simulink model "reconfig_dev_2021a_analytique"  (R2021a)
settings: Solver=VariableStepAuto  StartTime=0.0  StopTime=tsim  RelTol=1e-3
InitFcn:
  | main
values from neighbouring files (symbols this model uses):
  drone_params = get_parameters(3)    [main.m]
  dt = 0.005    [main.m]
  g = 9.81    [main.m]
  gust_duration = 5    [main.m]
  gust_force = [0;0;0]    [main.m]
  gust_start = 8    [main.m]
  omega0 = [[0,0,0]',[0,0,0]',[0,0,0]']    [main.m]
  p0 = [[0,0,2]',[0,0,2]',[0,0,2]']    [main.m]
  q0 = [[1,0,0,0]',[1,0,0,0]',[1,0,0,0]']    [main.m]
  tsim = 20    [main.m]
  v0 = [[0,0,0]',[0,0,0]',[0,0,0]']    [main.m]
undefined symbols (not defined in the file or in its folder): SMC_attitude_control, SMC_position_control, SMC_sliding_var, Twisting_attitude_control, Twisting_position_control, Twisting_sliding_var
libraries: vrlib x1
settings Model: Creator=gbattaglia2021  LastModifiedBy=jcolombini2021

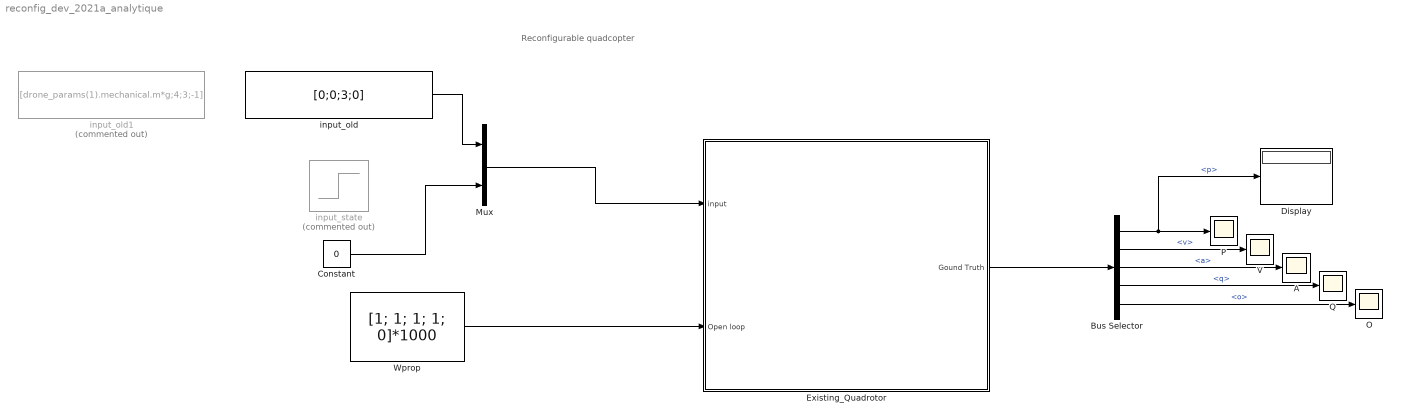
== system reconfig_dev_2021a_analytique ==
  note: Reconfigurable quadcopter
  "  Existing_Quadrotor" : Subsystem  mask{control_type_param=1: Position + Yaw, DroneID=1, DroneName=Drone1, idx_offset=0}
      mask prompts: control_type_param "Controller type"; DroneName "Drone Name"; idx_offset "Index Offset"
      mask TypeOptions control_type_param: 1: Position + Yaw | 2: Body Velocity + Yawrate | 3: Body Acceleration + Yawrate | 4: Thrust + Attitude | 5: Thrust + Body Rate | 6: Body Wrench
      mask TypeOptions DroneID: 1 | 2 | 3 | 4 | 5 | 6 | 7 | 8 | 9
      mask Callback DroneID:
      | ID = get_param(gcb,'DroneID');
      | offset = get_param(gcb,'idx_offset');
      | if ischar(ID)
      |   ID = str2num(ID);
      | end
      | if ischar(offset)
      |   offset = str2num(offset);
      | end
      | nameID = ID + offset;
      | set_param(gcb,'DroneName',["Drone"+num2str(nameID)]);
      mask Callback DroneName: set_param([gcb,'/To Workspace'],'VariableName',[get_param(gcb,'DroneName')]);
      mask Callback idx_offset:
      | ID = get_param(gcb,'DroneID');
      | offset = get_param(gcb,'idx_offset');
      | if ischar(ID)
      |   ID = str2num(ID);
      | end
      | if ischar(offset)
      |   offset = str2num(offset);
      | end
      | nameID = ID + offset;
      | set_param(gcb,'DroneName',["Drone"+num2str(nameID)]);
      mask DialogControl Control4 Prompt: click to choose controller
      mask Display:
      | image('format/drone_image.png'); % Use "Edit Image" on toolstrip to change.
      | Name = get_param(gcb,'DroneName');
      | ID = get_param(gcb,'DroneID');
      | C_mode = get_param(gcb,'control_type_param');
      | C_mode(1:2) = [];
      | color('red')
      | ID = "ID = "+ID;
      | color('red')
      | text(0.5, 0.25, Name, 'horizontalAlignment', 'center')
      | color('red')
      | text(0.5, 0.15, ID, 'horizontalAlignment', 'center')
      | color('blue');
      | text(0.5, 0.05, C_mode, 'horizontalAlignment', 'center')
  A : Scope
  Bus Selector : BusSelector  OutputSignals=p,v,a,q,o
  Constant : Constant  Value=0
  Display : Display
  Mux : Mux  Inputs=2
  O : Scope
  P : Scope
  Q : Scope
  V : Scope
  Wprop : Constant  Value=[1; 1; 1; 1; 0]*1000
  input_old : Constant  Value=[0;0;3;0]
  input_old1 : Constant  Commented=on  Value=[drone_params(1).mechanical.m*g;4;3;-1]
  input_state : Step  Commented=on  Time=tsim/2  Before=drone_params(1).control.state  After=drone_params(1).control.state_enum.folded2  SampleTime=0
  wires:
  Bus Selector/1 -> Display/1, P/1  "<p>"
  Bus Selector/4 -> Q/1  "<q>"
  Bus Selector/5 -> O/1  "<o>"
  Bus Selector/2 -> V/1  "<v>"
  "  Existing_Quadrotor"/1(Gound Truth) -> Bus Selector/1
  Bus Selector/3 -> A/1  "<a>"
  Wprop/1 -> "  Existing_Quadrotor"/2(Open loop)
  input_old/1 -> Mux/1
  Mux/1 -> "  Existing_Quadrotor"/1(input)
  Constant/1 -> Mux/2

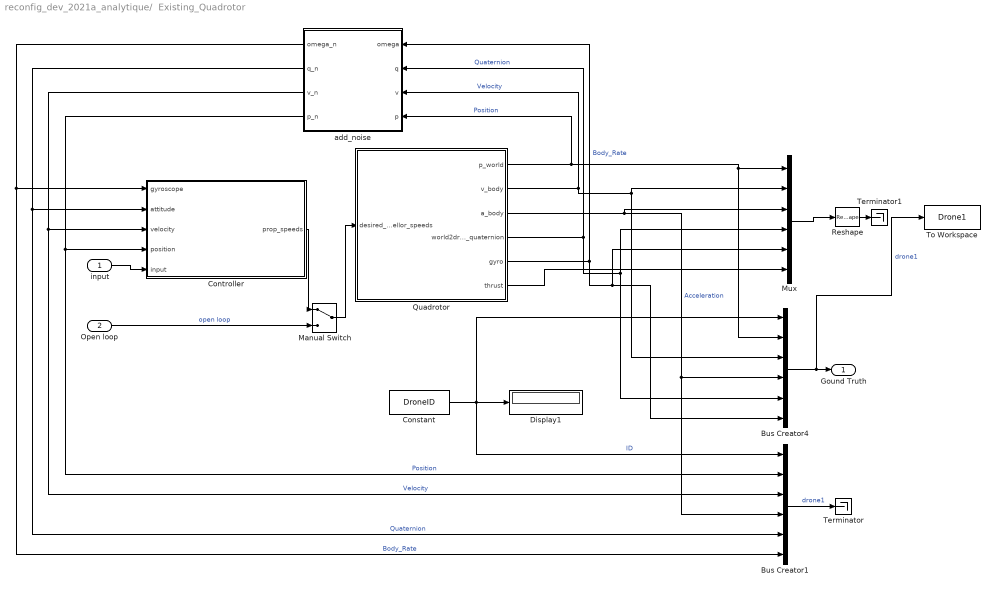
== system reconfig_dev_2021a_analytique/  Existing_Quadrotor ==
  input : Inport
  Open loop : Inport  Port=2
  Bus Creator1 : BusCreator  Inputs=6  OutDataTypeStr=Bus: DroneStateBus
      settings: InheritFromInputs=off
  Bus Creator4 : BusCreator  Inputs=6  OutDataTypeStr=Bus: DroneStateBus
      settings: InheritFromInputs=off
  Constant : Constant  Value=DroneID
  Controller : Subsystem
  Display1 : Display
  Manual Switch : ManualSwitch
  Mux : Mux  Inputs=6
  Quadrotor : Subsystem
      mask Display: image('droneHardware.jpeg'); % Use "Edit Image" on toolstrip to change.
  Reshape : Reshape
  Terminator : Terminator
  Terminator1 : Terminator
  To Workspace : ToWorkspace  VariableName=Drone1  SaveFormat=Timeseries  SampleTime=-1
  add_noise : MATLAB Function  TreatAsAtomicUnit=on
  Gound Truth : Outport
  wires:
  Quadrotor/5(gyro) -> add_noise/1(omega), Bus Creator4/6, Mux/5  "Body_Rate"
  Quadrotor/1(p_world) -> add_noise/4(p), Bus Creator4/2, Mux/1  "Position"
  Quadrotor/4(world2drone_quaternion) -> add_noise/2(q), Bus Creator4/5, Mux/4  "Quaternion"
  Mux/1 -> Reshape/1
  Quadrotor/2(v_body) -> add_noise/3(v), Bus Creator4/3, Mux/2  "Velocity"
  Quadrotor/6(thrust) -> Mux/6
  input/1 -> Controller/5(input)
  Bus Creator4/1 -> To Workspace/1, Gound Truth/1  "drone1"
  add_noise/2(q_n) -> Bus Creator1/5, Controller/2(attitude)  "Quaternion"
  Quadrotor/3(a_body) -> Mux/3, Bus Creator4/4, Bus Creator1/4  "Acceleration"
  Bus Creator1/1 -> Terminator/1  "drone1"
  add_noise/4(p_n) -> Bus Creator1/2, Controller/4(position)  "Position"
  add_noise/3(v_n) -> Bus Creator1/3, Controller/3(velocity)  "Velocity"
  Constant/1 -> Bus Creator4/1, Display1/1, Bus Creator1/1  "ID"
  add_noise/1(omega_n) -> Bus Creator1/6, Controller/1(gyroscope)  "Body_Rate"
  Reshape/1 -> Terminator1/1
  Manual Switch/1 -> Quadrotor/1(desired_propellor_speeds)
  Controller/1(prop_speeds) -> Manual Switch/1
  Open loop/1 -> Manual Switch/2  "open loop"

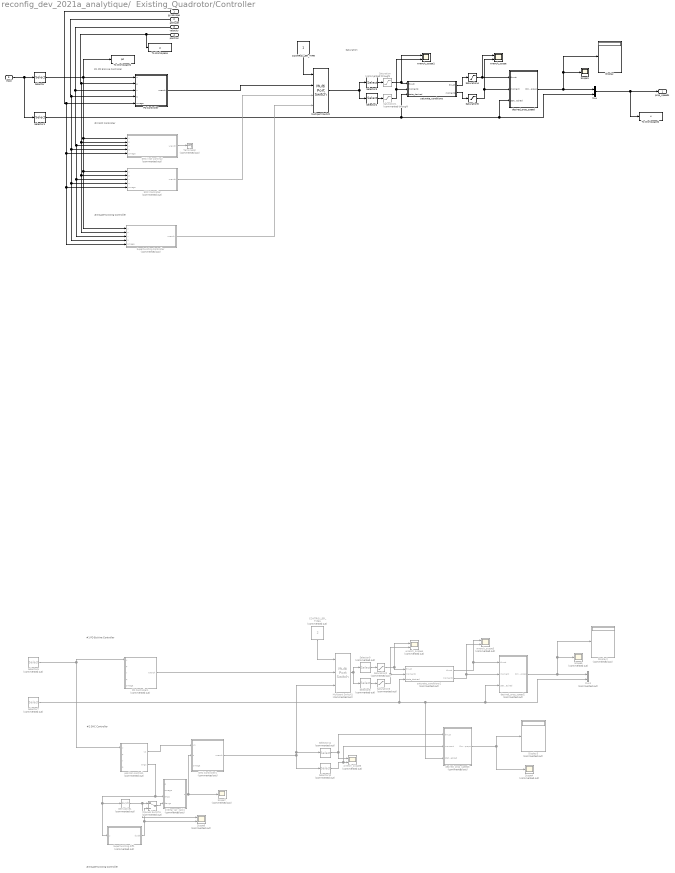
== system reconfig_dev_2021a_analytique/  Existing_Quadrotor/Controller ==
  note: Saturation
  note: #3 Supertwisting Controller
  note: #2 SMC Controller
  note: #1 PD Erskine Controller
  note: #3 Supertwisting Controller
  note: #1 PD Erskine Controller
  note: #2 SMC Controller
  gyroscope : Inport
  attitude : Inport  Port=2
  velocity : Inport  Port=3
  position : Inport  Port=4
  input : Inport  Port=5
  CONTROLLER_TYPE : Constant
  CONTROLLER_TYPE1 : Constant  Commented=on  Value=2
  Derivative1 : Derivative  Commented=on  CoefficientInTFapproximation=1000
  Display : Display
  Display2 : Display  Commented=on
  Display3 : Display  Commented=on
  Manual Switch1 : ManualSwitch  Commented=on
  Multiport Switch : MultiPortSwitch
  Multiport Switch1 : MultiPortSwitch  Commented=on  Inputs=2
  Mux : Mux  Inputs=2
  Mux1 : Mux  Commented=on  Inputs=2
  PD Controller : MATLAB Function  TreatAsAtomicUnit=on
  PD Controller1 : MATLAB Function  Commented=on  TreatAsAtomicUnit=on
  SMC (not working) : Subsystem  Commented=on
  SMC Controller : Subsystem  Commented=on
  SMC Controller1 : MATLAB Function  Commented=on  TreatAsAtomicUnit=on
  Saturation : Saturate  Commented=through  UpperLimit=16  LowerLimit=3
  Saturation1 : Saturate  Commented=through  UpperLimit=0.1  LowerLimit=-0.1
  Saturation2 : Saturate  Commented=on  UpperLimit=16  LowerLimit=3
  Saturation3 : Saturate  Commented=on  UpperLimit=0.1  LowerLimit=-0.1
  Saturation4 : Saturate  UpperLimit=16  LowerLimit=3
  Saturation5 : Saturate  UpperLimit=0.1  LowerLimit=-0.1
  Scope1 : Scope
  Scope4 : Scope  Commented=on
  Scope5 : Scope  Commented=on
  Scope6 : Scope  Commented=on  NumInputPorts=2
  Scope7 : Scope  Commented=on
  Selector : Selector  InputPortWidth=5  IndexOptions=Index vector (dialog)  Indices=[1 2 3 4]  OutputSizes=1
  Selector1 : Selector  InputPortWidth=5  IndexOptions=Index vector (dialog)  Indices=[5]  OutputSizes=1
  Selector10 : Selector  Commented=on  InputPortWidth=4  IndexOptions=Index vector (dialog)  Indices=[2 3 4]  OutputSizes=1
  Selector11 : Selector  Commented=on  InputPortWidth=4  IndexOptions=Index vector (dialog)  Indices=[1]  OutputSizes=1
  Selector2 : Selector  InputPortWidth=4  IndexOptions=Index vector (dialog)  Indices=[2 3 4]  OutputSizes=1
  Selector3 : Selector  InputPortWidth=4  IndexOptions=Index vector (dialog)  Indices=[1]  OutputSizes=1
  Selector6 : Selector  Commented=on  InputPortWidth=5  IndexOptions=Index vector (dialog)  Indices=[1 2 3 4]  OutputSizes=1
  Selector7 : Selector  Commented=on  InputPortWidth=5  IndexOptions=Index vector (dialog)  Indices=[5]  OutputSizes=1
  Selector8 : Selector  Commented=on  InputPortWidth=4  IndexOptions=Index vector (dialog)  Indices=[2 3 4]  OutputSizes=1
  Selector9 : Selector  Commented=on  InputPortWidth=4  IndexOptions=Index vector (dialog)  Indices=[1]  OutputSizes=1
  Supertwisting Controller : Subsystem  Commented=on
  Supertwisting diff1 : Subsystem  Commented=on
  Terminator : Terminator  Commented=on
  To Workspace : ToWorkspace  VariableName=p  SaveFormat=Timeseries  SampleTime=-1
  To Workspace1 : ToWorkspace  VariableName=pd  SaveFormat=Timeseries  SampleTime=-1
  To Workspace2 : ToWorkspace  VariableName=u  SaveFormat=Timeseries  SampleTime=-1
  desired_prop_speed : MATLAB Function  TreatAsAtomicUnit=on
  desired_prop_speed2 : MATLAB Function  Commented=on  TreatAsAtomicUnit=on
  desired_prop_speed3 : MATLAB Function  Commented=on  TreatAsAtomicUnit=on
  posiiton control1 : MATLAB Function  Commented=on  TreatAsAtomicUnit=on
  saturate_conditions : MATLAB Function  TreatAsAtomicUnit=on
  saturate_conditions1 : MATLAB Function  Commented=on  TreatAsAtomicUnit=on
  sliding_var_calc1 : MATLAB Function  Commented=on  TreatAsAtomicUnit=on
  wrench_scope : Scope  NumInputPorts=2
  wrench_scope1 : Scope  NumInputPorts=2
  wrench_scope3 : Scope  Commented=on  NumInputPorts=2
  wrench_scope4 : Scope  Commented=on  NumInputPorts=2
  wrench_scope5 : Scope  Commented=on  NumInputPorts=2
  prop_speeds : Outport
  wires:
  Saturation/1 -> wrench_scope1/1, saturate_conditions/1("thrust ")
  Saturation1/1 -> saturate_conditions/2("moments "), wrench_scope1/2
  Selector1/1 -> desired_prop_speed/3(state_desired), Mux/2, saturate_conditions/3(state_desired)
  input/1 -> Selector1/1, Selector/1
  Mux/1 -> To Workspace2/1, prop_speeds/1
  Selector2/1 -> Saturation1/1
  CONTROLLER_TYPE/1 -> Multiport Switch/1
  PD Controller/1(wrench) -> Multiport Switch/2
  Multiport Switch/1 -> Selector3/1, Selector2/1
  Selector3/1 -> Saturation/1
  desired_prop_speed/1(Omega_props) -> Mux/1, Scope1/1, Display/1
  Selector7/1 -> saturate_conditions1/3(state_desired), desired_prop_speed3/3(state_desired), desired_prop_speed2/3(state_desired), Mux1/2
  desired_prop_speed2/1(Omega_props) -> Mux1/1, Scope5/1, Display2/1
  Selector10/1 -> desired_prop_speed3/2(moment), wrench_scope5/2
  Manual Switch1/1 -> sliding_var_calc1/4(dangc)
  Selector11/1 -> wrench_scope5/1, desired_prop_speed3/1(thrust)
  CONTROLLER_TYPE1/1 -> Multiport Switch1/1
  Selector6/1 -> posiiton control1/1(u), PD Controller1/1(u)
  SMC Controller1/1(wrench) -> Selector10/1, Selector11/1, Multiport Switch1/3
  posiiton control1/2(angc) -> sliding_var_calc1/3(angc), Derivative1/1, Supertwisting diff1/1(u)
  Derivative1/1 -> Scope6/1, Manual Switch1/1
  PD Controller1/1(wrench) -> Multiport Switch1/2
  Multiport Switch1/1 -> Selector9/1, Selector8/1
  Selector8/1 -> Saturation3/1
  sliding_var_calc1/1(s) -> Scope7/1, SMC Controller1/2(s)
  Supertwisting diff1/1(du/dt) -> Manual Switch1/2, Scope6/2
  Saturation3/1 -> saturate_conditions1/2("moments "), wrench_scope4/2
  posiiton control1/1(u1) -> SMC Controller1/1(u1)
  Selector9/1 -> Saturation2/1
  desired_prop_speed3/1(Omega_props) -> Scope4/1, Display3/1
  Saturation2/1 -> wrench_scope4/1, saturate_conditions1/1("thrust ")
  saturate_conditions1/1(thrust) -> desired_prop_speed2/1(thrust), wrench_scope3/1
  saturate_conditions1/2(moments) -> desired_prop_speed2/2(moment), wrench_scope3/2
  saturate_conditions/2(moments) -> Saturation5/1
  Saturation4/1 -> wrench_scope/1, desired_prop_speed/1(thrust)
  Saturation5/1 -> wrench_scope/2, desired_prop_speed/2(moment)
  saturate_conditions/1(thrust) -> Saturation4/1
  Selector/1 -> To Workspace1/1, Supertwisting Controller/1(u), SMC Controller/1(u), SMC (not working)/1(u), PD Controller/1(u)
  gyroscope/1 -> PD Controller/5(omega), Supertwisting Controller/5(omega), SMC Controller/5(omega), SMC (not working)/5(omega)
  position/1 -> To Workspace/1, PD Controller/2(p), SMC (not working)/2(p), Supertwisting Controller/2(p), SMC Controller/2(p)
  velocity/1 -> PD Controller/3(v), Supertwisting Controller/3("v "), SMC Controller/3("v "), SMC (not working)/3(v)
  attitude/1 -> Supertwisting Controller/4(q), SMC Controller/4(q), SMC (not working)/4(q), PD Controller/4(q)
  SMC Controller/1(wrench) -> Multiport Switch/3
  Supertwisting Controller/1(wrench) -> Multiport Switch/4
  SMC (not working)/1(wrench) -> Terminator/1

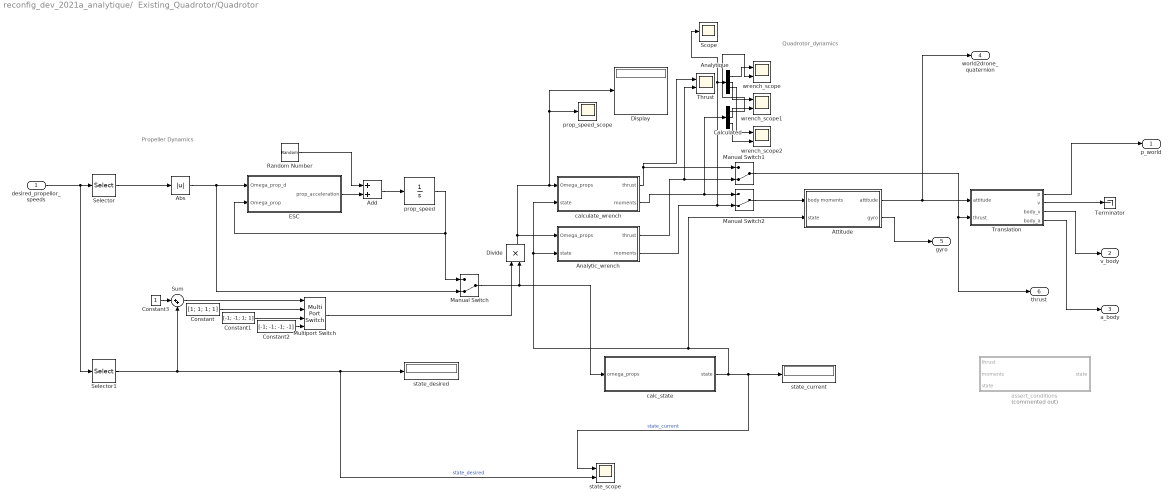
== system reconfig_dev_2021a_analytique/  Existing_Quadrotor/Quadrotor ==
  note: Quadrotor_dynamics
  note: Propeller Dynamics
  desired_propellor_speeds : Inport
  Abs : Abs
  Add : Sum
  Analytic_wrench : MATLAB Function  TreatAsAtomicUnit=on
  Analytique : Demux  Outputs=3
  Attitude : Subsystem
  Calculated : Demux  Outputs=3
  Constant : Constant  Value=[1; 1; 1; 1]
  Constant1 : Constant  Value=[-1; -1; 1; 1]
  Constant2 : Constant  Value=[-1; -1; -1; -1]
  Constant3 : Constant
  Display : Display
  Divide : Product
  ESC : MATLAB Function  TreatAsAtomicUnit=on
  Manual Switch : ManualSwitch  CurrentSetting=0
  Manual Switch1 : ManualSwitch  CurrentSetting=0
  Manual Switch2 : ManualSwitch  CurrentSetting=0
  Multiport Switch : MultiPortSwitch
  Random Number : RandomNumber  Mean=[0;0;0;0]  Variance=[5000;5000;5000;5000]  Seed=[1;2;3;4]  SampleTime=dt
  Scope : Scope
  Selector : Selector  InputPortWidth=5  IndexOptions=Index vector (dialog)  Indices=[1 2 3 4]  OutputSizes=1
  Selector1 : Selector  InputPortWidth=5  IndexOptions=Index vector (dialog)  Indices=[5]  OutputSizes=1
  Sum : Sum  Inputs=|++
  Terminator : Terminator
  Thrust : Scope  NumInputPorts=2
  Translation : Subsystem
  assert_conditions : MATLAB Function  Commented=on  TreatAsAtomicUnit=on
  calc_state : MATLAB Function  TreatAsAtomicUnit=on
  calculate_wrench : MATLAB Function  TreatAsAtomicUnit=on
  prop_speed : Integrator  InitialCondition=drone_params(DroneID).motors.omega0  LimitOutput=on  UpperSaturationLimit=drone_params(DroneID).motors.omega_max  LowerSaturationLimit=drone_params(DroneID).motors.omega_min
  prop_speed_scope : Scope
  state_current : Display
  state_desired : Display
  state_scope : Scope  NumInputPorts=2
  wrench_scope : Scope  NumInputPorts=2
  wrench_scope1 : Scope  NumInputPorts=2
  wrench_scope2 : Scope  NumInputPorts=2
  p_world : Outport
  v_body : Outport  Port=2
  a_body : Outport  Port=3
  world2drone_quaternion : Outport  Port=4
  gyro : Outport  Port=5
  thrust : Outport  Port=6
  wires:
  calculate_wrench/1(thrust) -> Thrust/1, Manual Switch1/1
  Add/1 -> prop_speed/1
  desired_propellor_speeds/1 -> Selector1/1, Selector/1
  prop_speed/1 -> Manual Switch/1, ESC/2(Omega_prop)
  calculate_wrench/2(moments) -> Manual Switch2/1, Calculated/1
  Attitude/1(attitude) -> world2drone_quaternion/1, Translation/1(attitude)
  Attitude/2(gyro) -> gyro/1
  Translation/3(body_v) -> v_body/1
  Translation/4(body_a) -> a_body/1
  Translation/1(p) -> p_world/1
  Random Number/1 -> Add/1
  ESC/1(prop_acceleration) -> Add/2
  Manual Switch/1 -> calc_state/1(omega_props), Divide/2
  Translation/2(v) -> Terminator/1
  Abs/1 -> Manual Switch/2, ESC/1(Omega_prop_d)
  Selector1/1 -> state_scope/2, state_desired/1, Sum/2  "state_desired"
  calc_state/1(state) -> state_scope/1, state_current/1, Analytic_wrench/2(state), calculate_wrench/2(state), Attitude/2(state)  "state_current"
  Selector/1 -> Abs/1
  Multiport Switch/1 -> Divide/1
  Divide/1 -> Analytic_wrench/1(Omega_props), Display/1, prop_speed_scope/1, calculate_wrench/1(Omega_props)
  Constant3/1 -> Sum/1
  Sum/1 -> Multiport Switch/1
  Constant/1 -> Multiport Switch/2
  Constant1/1 -> Multiport Switch/3
  Constant2/1 -> Multiport Switch/4
  Analytic_wrench/1(thrust) -> Manual Switch1/2, Thrust/2
  Analytic_wrench/2(moments) -> Manual Switch2/2, Scope/1, Analytique/1
  Manual Switch1/1 -> thrust/1, Translation/2(thrust)
  Manual Switch2/1 -> Attitude/1(body moments)
  Analytique/1 -> wrench_scope/1
  Analytique/3 -> wrench_scope2/1
  Analytique/2 -> wrench_scope1/1
  Calculated/1 -> wrench_scope/2
  Calculated/2 -> wrench_scope1/2
  Calculated/3 -> wrench_scope2/2

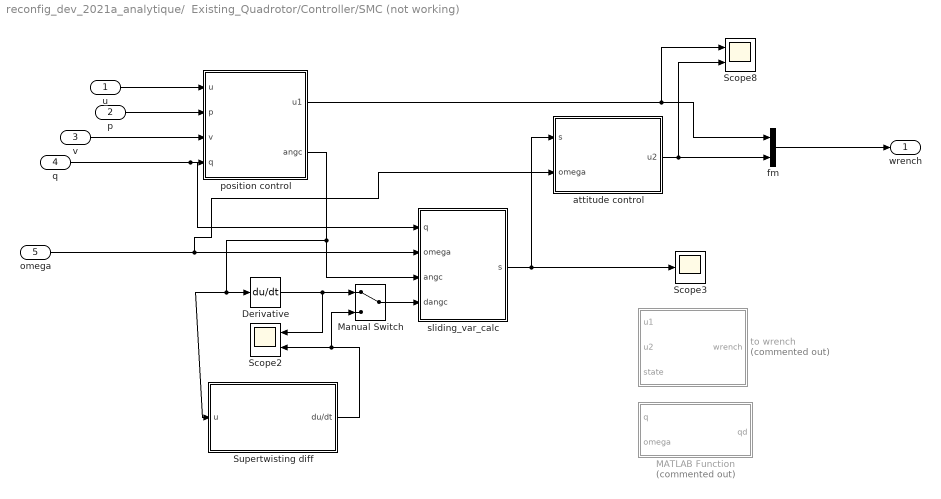
== system reconfig_dev_2021a_analytique/  Existing_Quadrotor/Controller/SMC (not working) ==
  u : Inport
  p : Inport  Port=2
  v : Inport  Port=3
  q : Inport  Port=4
  omega : Inport  Port=5
  Derivative : Derivative  CoefficientInTFapproximation=1000
  MATLAB Function : MATLAB Function  Commented=on  TreatAsAtomicUnit=on
  Manual Switch : ManualSwitch
  Scope2 : Scope  NumInputPorts=2
  Scope3 : Scope
  Scope8 : Scope  NumInputPorts=2
  Supertwisting diff : Subsystem
  attitude control : MATLAB Function  TreatAsAtomicUnit=on
  fm : Mux  Inputs=2
  position control : MATLAB Function  TreatAsAtomicUnit=on
  sliding_var_calc : MATLAB Function  TreatAsAtomicUnit=on
  to wrench : MATLAB Function  Commented=on  TreatAsAtomicUnit=on
  wrench : Outport
  wires:
  position control/2(angc) -> sliding_var_calc/3(angc), Supertwisting diff/1(u), Derivative/1
  position control/1(u1) -> fm/1, Scope8/1
  Supertwisting diff/1(du/dt) -> Manual Switch/2, Scope2/2
  Derivative/1 -> Manual Switch/1, Scope2/1
  q/1 -> position control/4(q), sliding_var_calc/1(q)
  attitude control/1(u2) -> fm/2, Scope8/2
  sliding_var_calc/1(s) -> Scope3/1, attitude control/1(s)
  v/1 -> position control/3(v)
  omega/1 -> attitude control/2(omega), sliding_var_calc/2(omega)
  Manual Switch/1 -> sliding_var_calc/4(dangc)
  fm/1 -> wrench/1
  p/1 -> position control/2(p)
  u/1 -> position control/1(u)

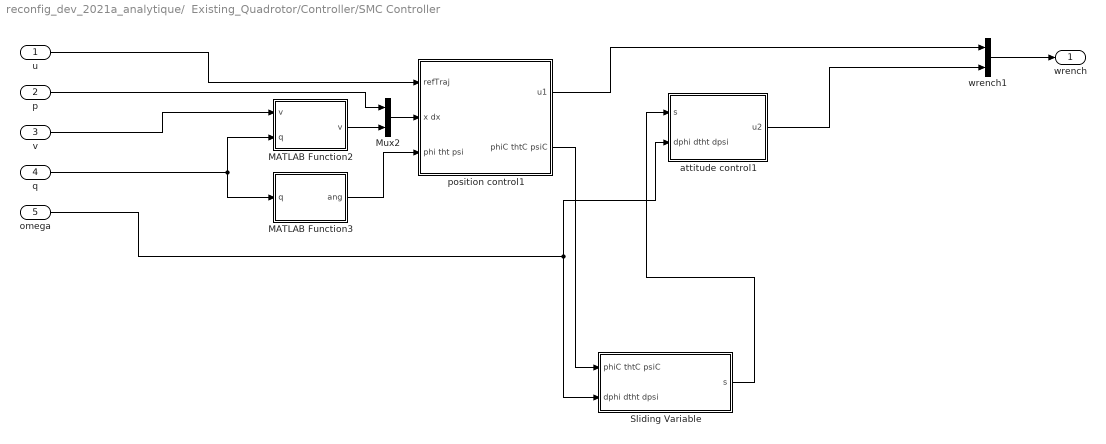
== system reconfig_dev_2021a_analytique/  Existing_Quadrotor/Controller/SMC Controller ==
  u : Inport
  p : Inport  Port=2
  "v " : Inport  Port=3
  q : Inport  Port=4
  omega : Inport  Port=5
  MATLAB Function2 : MATLAB Function  TreatAsAtomicUnit=on
  MATLAB Function3 : MATLAB Function  TreatAsAtomicUnit=on
  Mux2 : Mux  Inputs=2
  Sliding Variable : Subsystem
  attitude control1 : Subsystem
  position control1 : Subsystem
  wrench1 : Mux  Inputs=2
  wrench : Outport
  wires:
  position control1/2(phiC thtC psiC) -> Sliding Variable/1(phiC thtC psiC)
  q/1 -> MATLAB Function2/2(q), MATLAB Function3/1(q)
  p/1 -> Mux2/1
  attitude control1/1(u2) -> wrench1/2
  Sliding Variable/1(s) -> attitude control1/1(s)
  MATLAB Function2/1(v) -> Mux2/2
  Mux2/1 -> position control1/2(x dx)
  omega/1 -> attitude control1/2(dphi dtht dpsi), Sliding Variable/2(dphi dtht dpsi)
  position control1/1(u1) -> wrench1/1
  MATLAB Function3/1(ang) -> position control1/3(phi tht psi)
  wrench1/1 -> wrench/1
  u/1 -> position control1/1(refTraj)
  "v "/1 -> MATLAB Function2/1("v ")

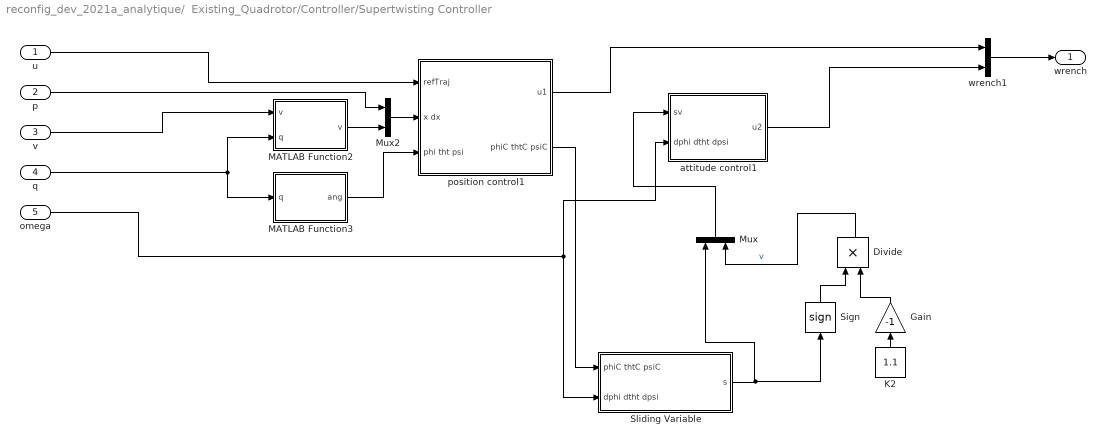
== system reconfig_dev_2021a_analytique/  Existing_Quadrotor/Controller/Supertwisting Controller ==
  u : Inport
  p : Inport  Port=2
  "v " : Inport  Port=3
  q : Inport  Port=4
  omega : Inport  Port=5
  Divide : Product
  Gain : Gain  Gain=-1
  K2 : Constant  Value=1.1
  MATLAB Function2 : MATLAB Function  TreatAsAtomicUnit=on
  MATLAB Function3 : MATLAB Function  TreatAsAtomicUnit=on
  Mux : Mux  Inputs=2
  Mux2 : Mux  Inputs=2
  Sign : Signum
  Sliding Variable : Subsystem
  attitude control1 : Subsystem
  position control1 : Subsystem
  wrench1 : Mux  Inputs=2
  wrench : Outport
  wires:
  position control1/2(phiC thtC psiC) -> Sliding Variable/1(phiC thtC psiC)
  q/1 -> MATLAB Function2/2(q), MATLAB Function3/1(q)
  p/1 -> Mux2/1
  attitude control1/1(u2) -> wrench1/2
  MATLAB Function2/1(v) -> Mux2/2
  Mux2/1 -> position control1/2(x dx)
  omega/1 -> attitude control1/2(dphi dtht dpsi), Sliding Variable/2(dphi dtht dpsi)
  position control1/1(u1) -> wrench1/1
  MATLAB Function3/1(ang) -> position control1/3(phi tht psi)
  wrench1/1 -> wrench/1
  u/1 -> position control1/1(refTraj)
  "v "/1 -> MATLAB Function2/1("v ")
  Sliding Variable/1(s) -> Sign/1, Mux/1
  Mux/1 -> attitude control1/1(sv)
  K2/1 -> Gain/1
  Sign/1 -> Divide/1
  Gain/1 -> Divide/2
  Divide/1 -> Mux/2  "v"

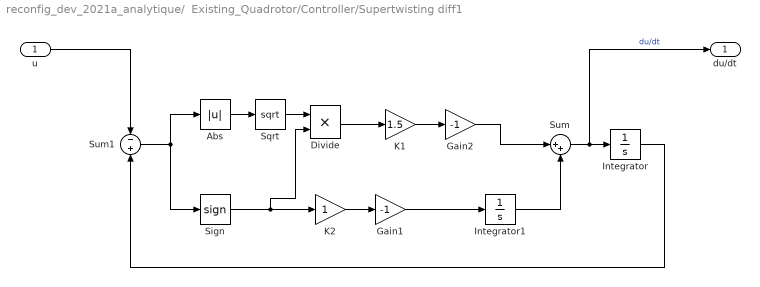
== system reconfig_dev_2021a_analytique/  Existing_Quadrotor/Controller/Supertwisting diff1 ==
  u : Inport
  Abs : Abs
  Divide : Product
  Gain1 : Gain  Gain=-1
  Gain2 : Gain  Gain=-1
  Integrator : Integrator  InitialCondition=[0;0;0]
  Integrator1 : Integrator  InitialCondition=[0;0;0]
  K1 : Gain  Gain=1.5
  K2 : Gain
  Sign : Signum
  Sqrt : Sqrt  SaturateOnIntegerOverflow=on
  Sum : Sum  Inputs=|++
  Sum1 : Sum  Inputs=-+
  du/dt : Outport
  wires:
  Integrator1/1 -> Sum/2
  Integrator/1 -> Sum1/2
  K1/1 -> Gain2/1
  Sum/1 -> du/dt/1, Integrator/1  "du/dt"
  Sum1/1 -> Sign/1, Abs/1
  Gain1/1 -> Integrator1/1
  K2/1 -> Gain1/1
  Abs/1 -> Sqrt/1
  Gain2/1 -> Sum/1
  Sign/1 -> Divide/2, K2/1
  Divide/1 -> K1/1
  Sqrt/1 -> Divide/1
  u/1 -> Sum1/1

== system reconfig_dev_2021a_analytique/  Existing_Quadrotor/Quadrotor/Attitude ==
  body moments : Inport
  state : Inport  Port=2
  Attitude : Integrator  InitialCondition=q0(:,DroneID)
  MATLAB Function : MATLAB Function  TreatAsAtomicUnit=on
  MATLAB Function1 : MATLAB Function  TreatAsAtomicUnit=on
  Normalize Vector : vrlib/Utilities/Normalize Vector  maxzero=0
  Sine Wave : Sin  Commented=on  Amplitude=[0.5;0.5;0.5]  Frequency=[1;0.3;0.6]  SampleTime=0
  angular velocity : Integrator  InitialCondition=omega0(:,DroneID)
  attitude : Outport
  gyro : Outport  Port=2
  wires:
  Attitude/1 -> Normalize Vector/1
  MATLAB Function/1(qd) -> Attitude/1  "quaternion derivative"
  body moments/1 -> MATLAB Function1/1(m)
  MATLAB Function1/1(a) -> angular velocity/1  "body angular acceleration"
  angular velocity/1 -> gyro/1, MATLAB Function/2(omega), MATLAB Function1/2(omega)  "gyroscope"
  Normalize Vector/1 -> MATLAB Function/1(q), attitude/1  "unit quaternion"
  state/1 -> MATLAB Function1/3(state)

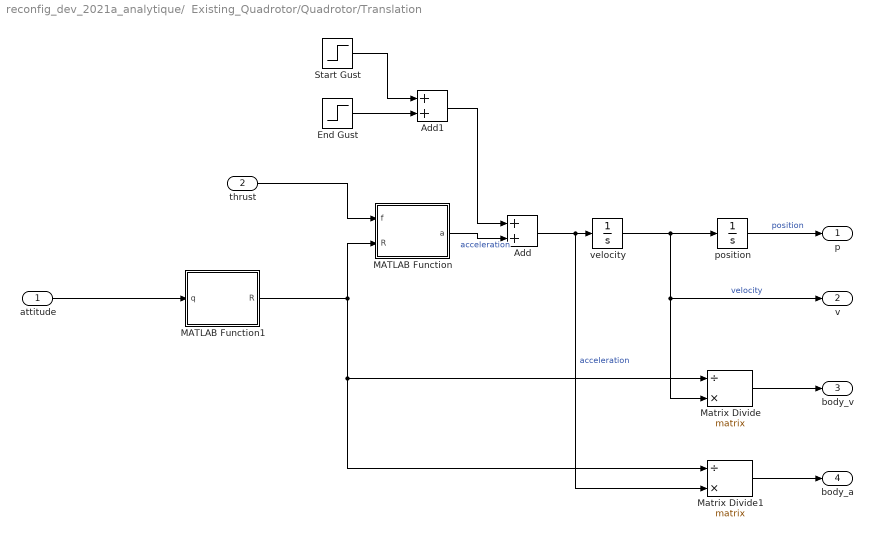
== system reconfig_dev_2021a_analytique/  Existing_Quadrotor/Quadrotor/Translation ==
  attitude : Inport
  thrust : Inport  Port=2
  Add : Sum
  Add1 : Sum
  End Gust : Step  Time=gust_start + gust_duration  Before=[0;0;0]  After=-1*gust_force/drone_params(DroneID).mechanical.m  SampleTime=0
  MATLAB Function : MATLAB Function  TreatAsAtomicUnit=on
  MATLAB Function1 : MATLAB Function  TreatAsAtomicUnit=on
  Matrix Divide : Product  Inputs=/*  Multiplication=Matrix(*)
  Matrix Divide1 : Product  Inputs=/*  Multiplication=Matrix(*)
  Start Gust : Step  Time=gust_start  Before=[0;0;0]  After=gust_force/drone_params(DroneID).mechanical.m  SampleTime=0
  position : Integrator  InitialCondition=p0(:,DroneID)
  velocity : Integrator  InitialCondition=v0(:,DroneID)
  p : Outport
  v : Outport  Port=2
  body_v : Outport  Port=3
  body_a : Outport  Port=4
  wires:
  velocity/1 -> Matrix Divide/2, v/1, position/1  "velocity"
  position/1 -> p/1  "position"
  Add/1 -> Matrix Divide1/2, velocity/1  "acceleration"
  attitude/1 -> MATLAB Function1/1(q)
  thrust/1 -> MATLAB Function/1(f)
  MATLAB Function1/1(R) -> Matrix Divide1/1, Matrix Divide/1, MATLAB Function/2(R)
  Matrix Divide/1 -> body_v/1
  Matrix Divide1/1 -> body_a/1
  MATLAB Function/1(a) -> Add/2  "acceleration"
  Add1/1 -> Add/1
  End Gust/1 -> Add1/2
  Start Gust/1 -> Add1/1

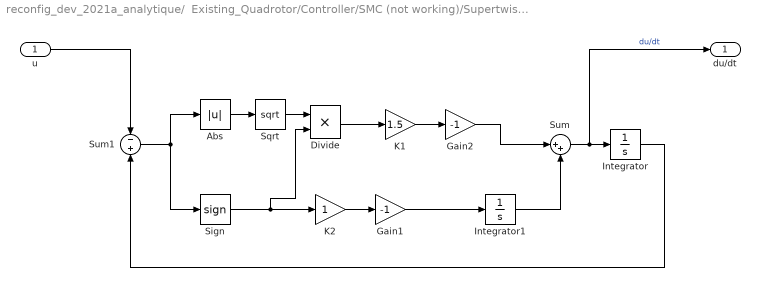
== system reconfig_dev_2021a_analytique/  Existing_Quadrotor/Controller/SMC (not working)/Supertwisting diff ==
  u : Inport
  Abs : Abs
  Divide : Product
  Gain1 : Gain  Gain=-1
  Gain2 : Gain  Gain=-1
  Integrator : Integrator  InitialCondition=[0;0;0]
  Integrator1 : Integrator  InitialCondition=[0;0;0]
  K1 : Gain  Gain=1.5
  K2 : Gain
  Sign : Signum
  Sqrt : Sqrt  SaturateOnIntegerOverflow=on
  Sum : Sum  Inputs=|++
  Sum1 : Sum  Inputs=-+
  du/dt : Outport
  wires:
  Integrator1/1 -> Sum/2
  Integrator/1 -> Sum1/2
  K1/1 -> Gain2/1
  Sum/1 -> du/dt/1, Integrator/1  "du/dt"
  Sum1/1 -> Sign/1, Abs/1
  Gain1/1 -> Integrator1/1
  K2/1 -> Gain1/1
  Abs/1 -> Sqrt/1
  Gain2/1 -> Sum/1
  Sign/1 -> Divide/2, K2/1
  Divide/1 -> K1/1
  Sqrt/1 -> Divide/1
  u/1 -> Sum1/1

== system reconfig_dev_2021a_analytique/  Existing_Quadrotor/Controller/SMC Controller/Sliding Variable ==
  phiC thtC psiC : Inport
  dphi dtht dpsi : Inport  Port=2
  Derivative : Derivative
  Integrator2 : Integrator
  Interpreted MATLAB Function : MATLABFcn  MATLABFcn=SMC_sliding_var(u)  OutputDimensions=3
  Mux2 : Mux
  s : Outport
  wires:
  Integrator2/1 -> Mux2/2
  Mux2/1 -> Interpreted MATLAB Function/1
  dphi dtht dpsi/1 -> Integrator2/1, Mux2/1
  Interpreted MATLAB Function/1 -> s/1
  phiC thtC psiC/1 -> Derivative/1, Mux2/3
  Derivative/1 -> Mux2/4

== system reconfig_dev_2021a_analytique/  Existing_Quadrotor/Controller/SMC Controller/attitude control1 ==
  s : Inport
  dphi dtht dpsi : Inport  Port=2
  Interpreted MATLAB Function : MATLABFcn  MATLABFcn=SMC_attitude_control(u)  OutputDimensions=3
  Mux : Mux  Inputs=2
  u2 : Outport
  wires:
  Mux/1 -> Interpreted MATLAB Function/1
  Interpreted MATLAB Function/1 -> u2/1
  dphi dtht dpsi/1 -> Mux/1
  s/1 -> Mux/2

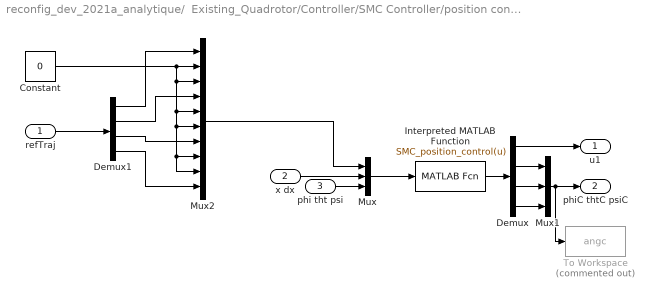
== system reconfig_dev_2021a_analytique/  Existing_Quadrotor/Controller/SMC Controller/position control1 ==
  refTraj : Inport
  x dx : Inport  Port=2
  phi tht psi : Inport  Port=3
  Constant : Constant  Value=0
  Demux : Demux
  Demux1 : Demux
  Interpreted MATLAB Function : MATLABFcn  MATLABFcn=SMC_position_control(u)  OutputDimensions=4
  Mux : Mux  Inputs=3
  Mux1 : Mux  Inputs=3
  Mux2 : Mux  Inputs=10
  To Workspace : ToWorkspace  Commented=on  VariableName=angc  SampleTime=-1
  u1 : Outport
  phiC thtC psiC : Outport  Port=2
  wires:
  Mux/1 -> Interpreted MATLAB Function/1
  x dx/1 -> Mux/2
  phi tht psi/1 -> Mux/3
  Interpreted MATLAB Function/1 -> Demux/1
  Demux/1 -> u1/1
  Demux/2 -> Mux1/1
  Demux/3 -> Mux1/2
  Demux/4 -> Mux1/3
  Mux1/1 -> To Workspace/1, phiC thtC psiC/1
  Mux2/1 -> Mux/1
  Constant/1 -> Mux2/9, Mux2/8, Mux2/6, Mux2/5, Mux2/3, Mux2/2
  refTraj/1 -> Demux1/1
  Demux1/1 -> Mux2/1
  Demux1/2 -> Mux2/4
  Demux1/3 -> Mux2/7
  Demux1/4 -> Mux2/10

== system reconfig_dev_2021a_analytique/  Existing_Quadrotor/Controller/Supertwisting Controller/Sliding Variable ==
  phiC thtC psiC : Inport
  dphi dtht dpsi : Inport  Port=2
  Derivative : Derivative
  Integrator2 : Integrator
  Interpreted MATLAB Function : MATLABFcn  MATLABFcn=Twisting_sliding_var(u)  OutputDimensions=3
  Mux2 : Mux
  s : Outport
  wires:
  Integrator2/1 -> Mux2/2
  Mux2/1 -> Interpreted MATLAB Function/1
  dphi dtht dpsi/1 -> Integrator2/1, Mux2/1
  Interpreted MATLAB Function/1 -> s/1
  phiC thtC psiC/1 -> Derivative/1, Mux2/3
  Derivative/1 -> Mux2/4

== system reconfig_dev_2021a_analytique/  Existing_Quadrotor/Controller/Supertwisting Controller/attitude control1 ==
  sv : Inport
  dphi dtht dpsi : Inport  Port=2
  Interpreted MATLAB Function : MATLABFcn  MATLABFcn=Twisting_attitude_control(u)  OutputDimensions=3
  Mux : Mux  Inputs=2
  u2 : Outport
  wires:
  Mux/1 -> Interpreted MATLAB Function/1
  Interpreted MATLAB Function/1 -> u2/1
  dphi dtht dpsi/1 -> Mux/1
  sv/1 -> Mux/2

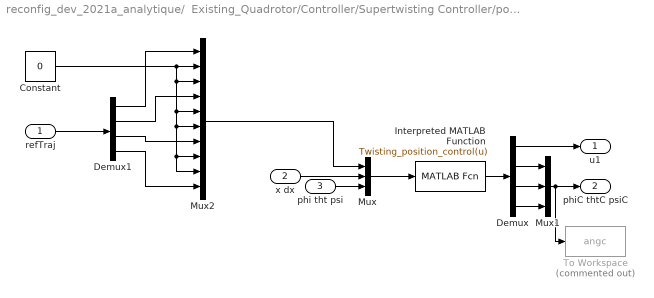
== system reconfig_dev_2021a_analytique/  Existing_Quadrotor/Controller/Supertwisting Controller/position control1 ==
  refTraj : Inport
  x dx : Inport  Port=2
  phi tht psi : Inport  Port=3
  Constant : Constant  Value=0
  Demux : Demux
  Demux1 : Demux
  Interpreted MATLAB Function : MATLABFcn  MATLABFcn=Twisting_position_control(u)  OutputDimensions=4
  Mux : Mux  Inputs=3
  Mux1 : Mux  Inputs=3
  Mux2 : Mux  Inputs=10
  To Workspace : ToWorkspace  Commented=on  VariableName=angc  SampleTime=-1
  u1 : Outport
  phiC thtC psiC : Outport  Port=2
  wires:
  Mux/1 -> Interpreted MATLAB Function/1
  x dx/1 -> Mux/2
  phi tht psi/1 -> Mux/3
  Interpreted MATLAB Function/1 -> Demux/1
  Demux/1 -> u1/1
  Demux/2 -> Mux1/1
  Demux/3 -> Mux1/2
  Demux/4 -> Mux1/3
  Mux1/1 -> To Workspace/1, phiC thtC psiC/1
  Mux2/1 -> Mux/1
  Constant/1 -> Mux2/9, Mux2/8, Mux2/6, Mux2/5, Mux2/3, Mux2/2
  refTraj/1 -> Demux1/1
  Demux1/1 -> Mux2/1
  Demux1/2 -> Mux2/4
  Demux1/3 -> Mux2/7
  Demux1/4 -> Mux2/10

== matlab function reconfig_dev_2021a_analytique/  Existing_Quadrotor/Controller/PD Controller1 ==
  data: u input; p input size=3; v input size=3; q input size=4; omega input size=3; wrench output size=4; control_type_param parameter; drone_params parameter; DroneID parameter; g parameter
function wrench = controller(u, p, v, q, omega, control_type_param, drone_params, DroneID, g)

    thrust = 1; % set output dim
    moments = [0;0;0]; % set output dim
    wrench = [0;0;0;0]; % set output dim

  coder.extrinsic('droneControl'); % link simulink to matlab function
  
  % do control
  [thrust, moments] = droneControl(u, p, v, q, omega, ...
    control_type_param, drone_params, DroneID, g);

  wrench = [thrust; moments];

end

== matlab function reconfig_dev_2021a_analytique/  Existing_Quadrotor/Controller/SMC Controller1 ==
  data: u1 input; s input size=3; omega input size=3; wrench output size=4; drone_params parameter; DroneID parameter
function wrench = controller(u1, s, omega, drone_params, DroneID)

%     thrust = 1; % set output dim
%     moments = [0;0;0]; % set output dim
    wrench = [0;0;0;0]; % set output dim

    coder.extrinsic('droneControlSMC'); % link simulink to matlab function
  
    % do control
    [thrust, moments] = droneControlSMC(u1, s, omega, ...
        drone_params, DroneID);

    wrench = [thrust; moments];

    
end

== matlab function reconfig_dev_2021a_analytique/  Existing_Quadrotor/Controller/desired_prop_speed2 ==
  data: thrust input; Omega_props output; moment input; state_desired input; drone_params parameter; DroneID parameter
function Omega_props  =  Allocation(thrust, moment, state_desired, drone_params, DroneID)

M = drone_params(DroneID).control.allocation_matrix;
if state_desired ~= drone_params(DroneID).control.state
switch state_desired
    case drone_params(DroneID).control.state_enum.unfolded
        M = drone_params(DroneID).control.allocation_matrix_u;
    case drone_params(DroneID).control.state_enum.folded2
        M = drone_params(DroneID).control.allocation_matrix_2f;
    case drone_params(DroneID).control.state_enum.folded4
        M = drone_params(DroneID).control.allocation_matrix_4f;
end
end

%  Omega_props = sqrt(inv(alloc_mat) * [thrust;moment]);
if state_desired ~= drone_params(DroneID).control.state_enum.folded4
    W2 = M \ [thrust;moment];
    Omega_props = real(sqrt(complex(W2)));
else
    W2 = pinv(M(2:4,:)) * moment;
    Omega_props = real(sqrt(complex(W2)));
end

if state_desired == drone_params(DroneID).control.state_enum.folded2
    Omega_props = Omega_props.*[-1; -1; 1; 1];
elseif state_desired == drone_params(DroneID).control.state_enum.folded4
    Omega_props = Omega_props.*[-1; -1; -1; -1];
end

== matlab function reconfig_dev_2021a_analytique/  Existing_Quadrotor/Controller/desired_prop_speed3 ==
  data: thrust input; Omega_props output; moment input; state_desired input; drone_params parameter; DroneID parameter
function Omega_props  =  Allocation(thrust, moment, state_desired, drone_params, DroneID)

M = drone_params(DroneID).control.allocation_matrix;
if state_desired ~= drone_params(DroneID).control.state
switch state_desired
    case drone_params(DroneID).control.state_enum.unfolded
        M = drone_params(DroneID).control.allocation_matrix_u;
    case drone_params(DroneID).control.state_enum.folded2
        M = drone_params(DroneID).control.allocation_matrix_2f;
    case drone_params(DroneID).control.state_enum.folded4
        M = drone_params(DroneID).control.allocation_matrix_4f;
end
end

%  Omega_props = sqrt(inv(alloc_mat) * [thrust;moment]);
if state_desired ~= drone_params(DroneID).control.state_enum.folded4
    W2 = M \ [thrust;moment];
    Omega_props = real(sqrt(complex(W2)));
else
    W2 = pinv(M(2:4,:)) * moment;
    Omega_props = real(sqrt(complex(W2)));
end

if state_desired == drone_params(DroneID).control.state_enum.folded2
    Omega_props = Omega_props.*[-1; -1; 1; 1];
elseif state_desired == drone_params(DroneID).control.state_enum.folded4
    Omega_props = Omega_props.*[-1; -1; -1; -1];
end

== matlab function reconfig_dev_2021a_analytique/  Existing_Quadrotor/Controller/posiiton control1 ==
  data: u input; u1 output size=1; p input; v input; q input; angc output size=3; g parameter; drone_params parameter; DroneID parameter
function [u1, angc] = SMCposcontrol(u,p,v,q,g, drone_params, DroneID)

u1 = 1;
angc = [0; 0; 0];
coder.extrinsic('SMCposition');

[u1, angc] = SMCposition(u,p,v,q,drone_params, DroneID,g);

== matlab function reconfig_dev_2021a_analytique/  Existing_Quadrotor/Controller/saturate_conditions1 ==
  data: thrust input; moments input; state_desired input; drone_params parameter; DroneID parameter; thrust output; moments output
function [thrust, moments] = saturate_conditions(thrust, moments, state_desired, drone_params, DroneID)

coder.extrinsic("solve_conditions");
coder.extrinsic("verify_conditions");
[verify_u, verify_2f] = verify_conditions(thrust,moments);

if state_desired == drone_params(DroneID).control.state_enum.unfolded
    if (verify_u)
        return;
    end
    moments(3) = solve_conditions(thrust,moments,"u");

elseif state_desired == drone_params(DroneID).control.state_enum.folded2
   if (~verify_u && verify_2f)
        return;
   end
   moments(3) = solve_conditions(thrust,moments,"2f");

elseif state_desired == drone_params(DroneID).control.state_enum.folded4
   if (~verify_u && ~verify_2f)
        return;
   end


end

== matlab function reconfig_dev_2021a_analytique/  Existing_Quadrotor/Controller/sliding_var_calc1 ==
  data: q input; s output; omega input; angc input; dangc input
function s=sliding_var(q, omega, angc, dangc)
s = [0; 0; 0]; ang = s;
% dang=[u(1);u(2);u(3)];
% ang=[u(4);u(5);u(6)];
% angc=[u(7);u(8);u(9)];
% dangc=[u(10);u(11);u(12)];
coder.extrinsic("quat2eul");
ang = quat2eul(q);
tuning_parameter = 100;
s=(omega-dangc)+tuning_parameter*(ang-angc);
end

== matlab function reconfig_dev_2021a_analytique/  Existing_Quadrotor/Controller/SMC (not working)/to wrench ==
  data: u1 input size=1; u2 input size=3; state input; wrench output size=4; drone_params parameter; DroneID parameter
function wrench  = allocator(u1, u2, state, drone_params, DroneID)

%     thrust = 1; % set output dim
%     moments = [0;0;0]; % set output dim
%     wrench = [0;0;0;0]; % set output dim
%     P = eye(4);
%     M = eye(4);

    wrench = [u1; u2];

%     if state == drone_params(DroneID).control.state_enum.unfolded
% %         P = drone_params(DroneID).control.ss_matrix_u;
%         M = drone_params(DroneID).control.allocation_matrix_u;
%     elseif state == drone_params(DroneID).control.state_enum.folded2
% %         P = drone_params(DroneID).control.ss_matrix_2f;
%         M = drone_params(DroneID).control.allocation_matrix_2f;
%     elseif state == drone_params(DroneID).control.state_enum.folded4
% %         P = drone_params(DroneID).control.ss_matrix_4f;
%         M = drone_params(DroneID).control.allocation_matrix_4f;
%     end
% 
% %     W2 = P \ U;
%     
%     wrench = M*W2;

    
end

== matlab function reconfig_dev_2021a_analytique/  Existing_Quadrotor/Controller/SMC (not working)/MATLAB Function ==
  data: q input size=4; omega input size=3; qd output size=4
function qd  = quaternion_derivative(q, omega)


qd =  0.5 * multiplyQuaternions([0;omega],q);

end


function q = multiplyQuaternions(qA,qB)
q0 = qA(1);
q1 = qA(2);
q2 = qA(3);
q3 = qA(4);
Q = [q0, -q1, -q2, -q3;
     q1,  q0, -q3,  q2;
     q2,  q3,  q0, -q1;
     q3, -q2,  q1,  q0];
q = Q * qB;
end

== matlab function reconfig_dev_2021a_analytique/  Existing_Quadrotor/Controller/Supertwisting Controller/MATLAB Function3 ==
  data: q input; ang output
function ang = q2e(q)

ang = quat2eul(q);

== matlab function reconfig_dev_2021a_analytique/  Existing_Quadrotor/Controller/SMC Controller/MATLAB Function2 ==
  data: v input; v output; q input
function v = fcn(v,q)

R = quat2rotm(q');

v = R*v;

== matlab function reconfig_dev_2021a_analytique/  Existing_Quadrotor/Controller/SMC Controller/MATLAB Function3 ==
  data: q input; ang output
function ang = q2e(q)

ang = quat2eul(q);

== matlab function reconfig_dev_2021a_analytique/  Existing_Quadrotor/Quadrotor/Analytic_wrench ==
  data: Omega_props input; state input; thrust output; moments output; drone_params parameter; DroneID parameter
function [thrust, moments] =  analyticAllocation(Omega_props, state, drone_params, DroneID)

t_motors = [zeros(2,4);
            (drone_params(DroneID).motors.kt_prop*Omega_props.^2).';
            zeros(2, 4);
            (drone_params(DroneID).motors.kd_prop*Omega_props.^2).']; %Thrust in motors frame

t_motors = t_motors(:,[3 1 4 2]);
        
switch state
    case drone_params(DroneID).control.state_enum.unfolded
        drone_params(DroneID).mechanical.Theta = drone_params.mechanical.Thetau;
    case drone_params(DroneID).control.state_enum.folded2
        drone_params(DroneID).mechanical.Theta  = drone_params(DroneID).mechanical.Theta2f;
    case drone_params(DroneID).control.state_enum.folded4
        drone_params(DroneID).mechanical.Theta = drone_params(DroneID).mechanical.Theta4f;
end

motor_to_hinge_r = zeros(3, 3);
t_body = zeros(3, 4);
m_body = zeros(3, 4);

for i = 1:4
    motor_to_hinge_r = Rymat(drone_params(DroneID).mechanical.Theta(i));
    t_body(:,i) = motor_to_hinge_r*t_motors(1:3,i); %transform motors frame to body frame
    motor_to_hinge_inbody = motor_to_hinge_r*drone_params.transforms.hinge_motor_p;
    motor_to_body_inbody = drone_params(DroneID).transforms.body_hinge_r(:,:,i)*motor_to_hinge_inbody + drone_params(DroneID).transforms.body_hinge_p(:,i);     m_from_t = cross(motor_to_body_inbody ,t_body(:,i));
    m_body(:,i) = (-1)^(i)*drone_params(DroneID).transforms.body_hinge_r(:,:,i)*motor_to_hinge_r*t_motors(4:6,i)+ m_from_t;

    %gambiarra em Z
%     m_body = m_body+ [0; 0; (-1)^(i)*t_motors(6,i)];
end


thrust_all = sum(t_body,2);
thrust = thrust_all(3);
moments = sum(m_body,2); % wrench(2:4);
moments(2) = -moments(2);

== matlab function reconfig_dev_2021a_analytique/  Existing_Quadrotor/Controller/PD Controller ==
  data: u input; p input size=3; v input size=3; q input size=4; omega input size=3; wrench output size=4; control_type_param parameter; drone_params parameter; DroneID parameter; g parameter
function wrench = controller(u, p, v, q, omega, control_type_param, drone_params, DroneID, g)
    thrust = 1; % set output dim
    moments = [0;0;0]; % set output dim
    wrench = [0;0;0;0]; % set output dim

  coder.extrinsic('droneControl'); % link simulink to matlab function
  
  % do control
  [thrust, moments] = droneControl(u, p, v, q, omega, ...
    control_type_param, drone_params, DroneID, g);

  wrench = [thrust; moments];

end

== matlab function reconfig_dev_2021a_analytique/  Existing_Quadrotor/Controller/desired_prop_speed ==
  data: thrust input; Omega_props output; moment input; state_desired input; drone_params parameter; DroneID parameter
function Omega_props  =  Allocation(thrust, moment, state_desired, drone_params, DroneID)

M = drone_params(DroneID).control.allocation_matrix;
if state_desired ~= drone_params(DroneID).control.state
switch state_desired
    case drone_params(DroneID).control.state_enum.unfolded
        M = drone_params(DroneID).control.allocation_matrix_u;
    case drone_params(DroneID).control.state_enum.folded2
        M = drone_params(DroneID).control.allocation_matrix_2f;
    case drone_params(DroneID).control.state_enum.folded4
        M = drone_params(DroneID).control.allocation_matrix_4f;
end
end

%  Omega_props = sqrt(inv(alloc_mat) * [thrust;moment]);
if state_desired ~= drone_params(DroneID).control.state_enum.folded4
    W2 = M \ [thrust;moment];
    Omega_props = real(sqrt(complex(W2)));
else
    W2 = pinv(M(2:4,:)) * moment;
    Omega_props = real(sqrt(complex(W2)));
end

if state_desired == drone_params(DroneID).control.state_enum.folded2
    Omega_props = Omega_props.*[-1; -1; 1; 1];
elseif state_desired == drone_params(DroneID).control.state_enum.folded4
    Omega_props = Omega_props.*[-1; -1; -1; -1];
end

== matlab function reconfig_dev_2021a_analytique/  Existing_Quadrotor/Controller/saturate_conditions ==
  data: thrust input; moments input; state_desired input; drone_params parameter; DroneID parameter; thrust output; moments output
function [thrust, moments] = saturate_conditions(thrust, moments, state_desired, drone_params, DroneID)

coder.extrinsic("solve_conditions");
coder.extrinsic("verify_conditions");
[verify_u, verify_2f] = verify_conditions(thrust,moments);

if state_desired == drone_params(DroneID).control.state_enum.unfolded
    if (verify_u)
        return;
    end
    moments(3) = solve_conditions(thrust,moments,"u");

elseif state_desired == drone_params(DroneID).control.state_enum.folded2
   if (~verify_u && verify_2f)
        return;
   end
   moments(3) = solve_conditions(thrust,moments,"2f");

elseif state_desired == drone_params(DroneID).control.state_enum.folded4
   if (~verify_u && ~verify_2f)
        return;
   end


end

== matlab function reconfig_dev_2021a_analytique/  Existing_Quadrotor/Quadrotor/Attitude/MATLAB Function ==
  data: q input size=4; omega input size=3; qd output size=4
function qd  = quaternion_derivative(q, omega)


qd =  0.5 * multiplyQuaternions([0;omega],q);

end


function q = multiplyQuaternions(qA,qB)
q0 = qA(1);
q1 = qA(2);
q2 = qA(3);
q3 = qA(4);
Q = [q0, -q1, -q2, -q3;
     q1,  q0, -q3,  q2;
     q2,  q3,  q0, -q1;
     q3, -q2,  q1,  q0];
q = Q * qB;
end

== matlab function reconfig_dev_2021a_analytique/  Existing_Quadrotor/Quadrotor/Attitude/MATLAB Function1 ==
  data: m input; a output; omega input; state input; drone_params parameter; DroneID parameter
function a = moments2angularacceleration(m, omega, state, drone_params, DroneID)

I = drone_params(DroneID).mechanical.I;
switch state
    case drone_params(DroneID).control.state_enum.unfolded
        I = drone_params(DroneID).mechanical.Iu;
    case drone_params(DroneID).control.state_enum.folded2
        I = drone_params(DroneID).mechanical.I2f;
    case drone_params(DroneID).control.state_enum.folded4
        I = drone_params(DroneID).mechanical.I4f;
end

a = inv(I)*m  - inv(I) * cross(omega,I*omega);

== matlab function reconfig_dev_2021a_analytique/  Existing_Quadrotor/Quadrotor/ESC ==
  data: Omega_prop_d input; prop_acceleration output; Omega_prop input; DroneID parameter; drone_params parameter
function prop_acceleration  =  ESC_ctrl(Omega_prop_d, Omega_prop, DroneID, drone_params)

prop_acceleration = (Omega_prop_d - Omega_prop)*drone_params(DroneID).motors.gain;

== matlab function reconfig_dev_2021a_analytique/  Existing_Quadrotor/Quadrotor/Translation/MATLAB Function ==
  data: f input; a output; R input; g parameter; drone_params parameter; DroneID parameter
function a = fcn(f, R, g, drone_params, DroneID)
m = drone_params(DroneID).mechanical.m;
a = R*[0;0;f]/m - [0;0;g];

== matlab function reconfig_dev_2021a_analytique/  Existing_Quadrotor/Quadrotor/Translation/MATLAB Function1 ==
  data: q input; R output
function R = quat2rotm(q)
  R = eye(3);
  coder.extrinsic('quat2rotm.m');
  R = quat2rotm(q);
end

== matlab function reconfig_dev_2021a_analytique/  Existing_Quadrotor/Quadrotor/calculate_wrench ==
  data: Omega_props input; state input; thrust output; moments output; drone_params parameter; DroneID parameter
function [thrust, moments] =  invAllocation(Omega_props, state, drone_params, DroneID)

M = drone_params(DroneID).control.allocation_matrix;
if state ~= drone_params(DroneID).control.state
switch state
    case drone_params(DroneID).control.state_enum.unfolded
        M = drone_params(DroneID).control.allocation_matrix_u;
    case drone_params(DroneID).control.state_enum.folded2
        M = drone_params(DroneID).control.allocation_matrix_2f;
    case drone_params(DroneID).control.state_enum.folded4
        M = drone_params(DroneID).control.allocation_matrix_4f;
end
end

wrench = M*(Omega_props.^2);

thrust = wrench(1);
moments = wrench(2:4);

== matlab function reconfig_dev_2021a_analytique/  Existing_Quadrotor/add_noise ==
  settings: updateMethod=DISCRETE
  data: omega input; omega_n output size=3; q input; v input; p input; q_n output size=4; v_n output size=3; p_n output size=3; drone_params parameter; DroneID parameter
function [omega_n, q_n, v_n, p_n]= add_noise(omega,q,v,p, drone_params, DroneID)

omega_n = omega + drone_params(DroneID).sensor.gyroscope_noise*(rand(3,1)-0.5);

q_n = q + drone_params(DroneID).sensor.attitude_noise*(rand(4,1)-0.5);
q_n = q_n/norm(q_n);

v_n = v + drone_params(DroneID).sensor.velocity_noise*(rand(3,1)-0.5);

p_n = p + drone_params(DroneID).sensor.position_noise*(rand(3,1)-0.5);

end

== matlab function reconfig_dev_2021a_analytique/  Existing_Quadrotor/Quadrotor/calc_state ==
  data: omega_props input; drone_params parameter; DroneID parameter; state output
function state = calculate_state(omega_props, drone_params, DroneID)

omega_indicator = omega_props >= 0;

if sum(omega_indicator) == 4
%     disp("Passing to u");
    state = drone_params(DroneID).control.state_enum.unfolded;
elseif sum(omega_indicator) == 2
%     disp("Passing to 2f");
    state = drone_params(DroneID).control.state_enum.folded2;
else
%     disp("Passing to 4f");
    state = drone_params(DroneID).control.state_enum.folded4;
% else
%     disp("WARNING: not possible condition");
%     state = drone_params(DroneID).control.state_enum.unfolded;
end

== matlab function reconfig_dev_2021a_analytique/  Existing_Quadrotor/Controller/SMC (not working)/attitude control ==
  data: s input; omega input size=3; u2 output size=3; drone_params parameter; DroneID parameter
function u2 = controller(s, omega, drone_params, DroneID)

%     thrust = 1; % set output dim
%     moments = [0;0;0]; % set output dim
    u2 = [0;0;0]; % set output dim

    coder.extrinsic('droneControlSMC'); % link simulink to matlab function
  
    % do control
    u2 = droneControlSMC(s, omega, ...
        drone_params, DroneID);

%     wrench = [thrust; moments];

    
end

== matlab function reconfig_dev_2021a_analytique/  Existing_Quadrotor/Controller/SMC (not working)/position control ==
  data: u input; u1 output size=1; p input; v input; q input; angc output size=3; g parameter; drone_params parameter; DroneID parameter
function [u1, angc] = SMCposcontrol(u,p,v,q,g, drone_params, DroneID)

u1 = 1;
angc = [0; 0; 0];
coder.extrinsic('SMCposition');

[u1, angc] = SMCposition(u,p,v,q,drone_params, DroneID,g);

== matlab function reconfig_dev_2021a_analytique/  Existing_Quadrotor/Quadrotor/assert_conditions ==
  data: thrust input; moments input; state input; drone_params parameter; DroneID parameter; state output
function state = assert_conditions(thrust, moments, state, drone_params, DroneID)

coder.extrinsic("verify_conditions");
[verify_u,verify_2f] = verify_conditions(thrust,moments);

if state == drone_params(DroneID).control.state_enum.unfolded
    if verify_u
       return;
    elseif verify_2f
        disp("Passing to 2f");
        drone_params(DroneID).mechanical.I = drone_params(DroneID).mechanical.I2f;
        state = drone_params(DroneID).control.state_enum.folded2;
%         drone_params(DroneID).control.allocation_matrix = drone_params(DroneID).control.allocation_matrix_2f;
    else
        disp("Passing to 4f");
        drone_params(DroneID).mechanical.I = drone_params(DroneID).mechanical.I4f;
        state = drone_params(DroneID).control.state_enum.folded4;
%         drone_params(DroneID).control.allocation_matrix = drone_params(DroneID).control.allocation_matrix_4f;
    end
elseif state == drone_params(DroneID).control.state_enum.folded2
    if verify_u
       disp("Passing to u");
       drone_params(DroneID).mechanical.I = drone_params(DroneID).mechanical.Iu;
       state = drone_params(DroneID).control.state_enum.unfolded;
%        drone_params(DroneID).control.allocation_matrix = drone_params(DroneID).control.allocation_matrix_u;
    elseif verify_2f
        return;
    else
        disp("Passing to 4f");
        drone_params(DroneID).mechanical.I = drone_params(DroneID).mechanical.I4f;
        state = drone_params(DroneID).control.state_enum.folded4;
%         drone_params(DroneID).control.allocation_matrix = drone_params(DroneID).control.allocation_matrix_4f;
    end
elseif state == drone_params(DroneID).control.state_enum.folded4
    if verify_u
        disp("Passing to u");
        drone_params(DroneID).mechanical.I = drone_params(DroneID).mechanical.Iu;
        drone_params(DroneID).control.state = drone_params(DroneID).control.state_enum.unfolded;
%         drone_params(DroneID).control.allocation_matrix = drone_params(DroneID).control.allocation_matrix_u;
    elseif verify_2f
        disp("Passing to 2f");
        drone_params(DroneID).mechanical.I = drone_params(DroneID).mechanical.I2f;
        state = drone_params(DroneID).control.state_enum.folded2;
%         drone_params(DroneID).control.allocation_matrix = drone_params(DroneID).control.allocation_matrix_2f;
    else
       return; 
    end
end

== matlab function reconfig_dev_2021a_analytique/  Existing_Quadrotor/Controller/SMC (not working)/sliding_var_calc ==
  data: q input; s output; omega input; angc input; dangc input
function s=sliding_var(q, omega, angc, dangc)
s = [0; 0; 0]; ang = s;
% dang=[u(1);u(2);u(3)];
% ang=[u(4);u(5);u(6)];
% angc=[u(7);u(8);u(9)];
% dangc=[u(10);u(11);u(12)];
coder.extrinsic("quat2eul");
ang = quat2eul(q);
% angc = quat2eul(qc);
tuning_parameter = 100;
s=(omega-dangc)+tuning_parameter*(ang-angc);
end

== matlab function reconfig_dev_2021a_analytique/  Existing_Quadrotor/Controller/Supertwisting Controller/MATLAB Function2 ==
  data: v input; v output; q input
function v = fcn(v,q)

R = quat2rotm(q');

v = R*v;
